simulink model "rtwdemo_stateflow_leg_code"  (Simulink 7.1)
settings: Solver=FixedStepDiscrete  StartTime=0.0  StopTime=10.0  RelTol=1e-3
PostLoadFcn:
  | load legcodeadder.mat;
settings Model: Creator=ajayaram  LastModifiedBy=ajayaram
settings SolverCC: AutoInsertRateTranBlk=on
settings DataIOCC: SaveOutput=off  SaveTime=off
settings OptimizationCC: InlineParams=on  InlineInvariantSignals=on  EnforceIntegerDowncast=off  StateBitsets=on  DataBitsets=on  UseTempVars=on  OptimizeModelRefInitCode=on  LifeSpan=1
settings DebuggingCC: SignalResolutionControl=TryResolveAll
settings RTWCC: SystemTargetFile=ert.tlc  TemplateMakefile=ert_default_tmf  Description=Real-Time Workshop Embedded Coder (no auto configuration)  GenerateReport=on  RTWVerbose=off  ProcessScript=ert_make_rtw_hook  CustomHeaderCode="#include \"add.h\""  CustomSource=add.c  IncludeHyperlinkInReport=on  LaunchReport=on
settings CodeAppCC: IgnoreCustomStorageClasses=off  CustomSymbolStrGlobalVar=rt$N$M  CustomSymbolStrType=$N$M  CustomSymbolStrFcn=$N$M$F  CustomSymbolStrMacro=$N$M
settings ERTTargetCC: GenerateSampleERTMain=on  SuppressErrorStatus=on  SupportAbsoluteTime=off  SupportNonFinite=off  SupportComplex=off  InlinedParameterPlacement=NonHierarchical  RootIOFormat=Structure reference  ERTCustomFileTemplate=example_file_process.tlc

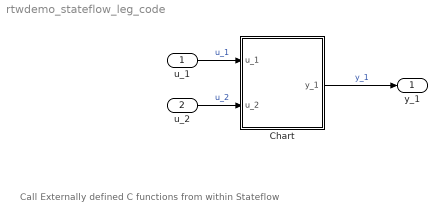
== system rtwdemo_stateflow_leg_code ==
  note: Call Externally defined C functions from within Stateflow
  u_1 : Inport  OutDataType=sfix(16)  OutScaling=2^0
  u_2 : Inport  Port=2  OutDataType=sfix(16)  OutScaling=2^0
  Chart : Stateflow chart
  y_1 : Outport  OutDataType=sfix(16)  OutScaling=2^0
  wires:
  u_1/1 -> Chart/1(u_1)  "u_1"
  u_2/1 -> Chart/2(u_2)  "u_2"
  Chart/1(y_1) -> y_1/1  "y_1"

== stateflow chart Chart ==
  (default) -> (junction 3)
  (junction 3) -> (junction 4) : {
      | y_1 = add(u_1,u_2) ;
      | }
  data: u_1 input double; u_2 input double; y_1 output double
